simulink model "IEEE30_case"  (R2024b)
settings: Solver=FixedStepAuto  StartTime=0  StopTime=5  FixedStep=1e-7  RelTol=1e-3
values from neighbouring files (symbols this model uses):
  GFL_DFIG_7_C_bus = 0.08    [IEEE30_case_parameters.m]
  GFL_DFIG_7_D_mutual = 2.500000e+3    (= 2500)    [IEEE30_case_parameters.m]
  GFL_DFIG_7_f0 = 60    [IEEE30_case_parameters.m]
  GFL_DFIG_7_gPLLi = 3200    [IEEE30_case_parameters.m]
  GFL_DFIG_7_gPLLp = 650    [IEEE30_case_parameters.m]
  GFL_DFIG_7_H_WT = 0.4    [IEEE30_case_parameters.m]
  GFL_DFIG_7_Hg = 0.8    [IEEE30_case_parameters.m]
  GFL_DFIG_7_Igq_ref = 0    [IEEE30_case_parameters.m]
  GFL_DFIG_7_Ird_ref = 704.45696    [IEEE30_case_parameters.m]
  GFL_DFIG_7_KI_V = -300000    [IEEE30_case_parameters.m]
  GFL_DFIG_7_KP_V = -1000    [IEEE30_case_parameters.m]
  GFL_DFIG_7_Ksh = 1.254300e+4    (= 12543)    [IEEE30_case_parameters.m]
  GFL_DFIG_7_Lg = 0.000483    [IEEE30_case_parameters.m]
  GFL_DFIG_7_Lm_pu = 4    [IEEE30_case_parameters.m]
  GFL_DFIG_7_N = 100    [IEEE30_case_parameters.m]
  GFL_DFIG_7_p = 2    [IEEE30_case_parameters.m]
  GFL_DFIG_7_Pitch = 0    [IEEE30_case_parameters.m]
  GFL_DFIG_7_R = 44    [IEEE30_case_parameters.m]
  GFL_DFIG_7_Rg = 2.000000e-5    (= 2e-05)    [IEEE30_case_parameters.m]
  GFL_DFIG_7_rho = 1.225    [IEEE30_case_parameters.m]
  GFL_DFIG_7_rPLLi = 4500    [IEEE30_case_parameters.m]
  GFL_DFIG_7_rPLLp = 620    [IEEE30_case_parameters.m]
  GFL_DFIG_7_Rs_pu = 0.011    [IEEE30_case_parameters.m]
  GFL_DFIG_7_Sbase = 2.000000e+6    (= 2000000)    [IEEE30_case_parameters.m]
  GFL_DFIG_7_ugq_ref = 0    [IEEE30_case_parameters.m]
  GFL_DFIG_7_usd_ref = 0    [IEEE30_case_parameters.m]
  GFL_DFIG_7_Vbase = 690    [IEEE30_case_parameters.m]
  GFL_DFIG_7_Vdc_ref = 1200    [IEEE30_case_parameters.m]
  GFL_DFIG_7_wind = 12    [IEEE30_case_parameters.m]
  GFL_DFIG_7_wm_ref = 518.184209    [IEEE30_case_parameters.m]
  SG_D_13_D = 0.01056    [IEEE30_case_parameters.m]
  SG_D_13_EnableSaturation = 0    [IEEE30_case_parameters.m]
  SG_D_13_f0 = 60    [IEEE30_case_parameters.m]
  SG_D_13_H = 7.5    [IEEE30_case_parameters.m]
  SG_D_13_K_A = 20    [IEEE30_case_parameters.m]
  SG_D_13_K_E = 1.000000e+1    (= 10)    [IEEE30_case_parameters.m]
  SG_D_13_K_F = 2.363    [IEEE30_case_parameters.m]
  SG_D_13_K_s = 0.5    [IEEE30_case_parameters.m]
  SG_D_13_R_a = 0.001088    [IEEE30_case_parameters.m]
  SG_D_13_S_A = 1    [IEEE30_case_parameters.m]
  SG_D_13_S_B = 0.103    [IEEE30_case_parameters.m]
  SG_D_13_S_N = 10.659857    [IEEE30_case_parameters.m]
  SG_D_13_SpeedPara = 200    [IEEE30_case_parameters.m]
  SG_D_13_T_0 = 0.370163    [IEEE30_case_parameters.m]
  SG_D_13_T_1 = 0.3    [IEEE30_case_parameters.m]
  SG_D_13_T_2 = 0.05    [IEEE30_case_parameters.m]
  SG_D_13_T_3 = 0.02    [IEEE30_case_parameters.m]
  SG_D_13_T_4 = 0.005    [IEEE30_case_parameters.m]
  SG_D_13_T_A = 0.02    [IEEE30_case_parameters.m]
  SG_D_13_T_dd = 8.000000e+0    (= 8)    [IEEE30_case_parameters.m]
  SG_D_13_T_ddd = 0.04    [IEEE30_case_parameters.m]
  SG_D_13_T_E = 0.314    [IEEE30_case_parameters.m]
  SG_D_13_T_F = 0.35    [IEEE30_case_parameters.m]
  SG_D_13_T_qd = 0.8    [IEEE30_case_parameters.m]
  SG_D_13_T_qdd = 0.02    [IEEE30_case_parameters.m]
  SG_D_13_T_speed = 0.1    [IEEE30_case_parameters.m]
  SG_D_13_T_w = 0.5    [IEEE30_case_parameters.m]
  SG_D_13_V_ref = 1.696619    [IEEE30_case_parameters.m]
  SG_D_13_w_ref = 376.991118    [IEEE30_case_parameters.m]
  SG_D_13_x_d = 1.9    [IEEE30_case_parameters.m]
  SG_D_13_x_dd = 0.302    [IEEE30_case_parameters.m]
  SG_D_13_x_ddd = 0.204    [IEEE30_case_parameters.m]
  SG_D_13_x_l = 0.05    [IEEE30_case_parameters.m]
  SG_D_13_x_q = 1.3    [IEEE30_case_parameters.m]
  SG_D_13_x_qd = 0.5    [IEEE30_case_parameters.m]
  SG_D_13_x_qdd = 0.3    [IEEE30_case_parameters.m]
  SG_D_1_D = 0.01056    [IEEE30_case_parameters.m]
  SG_D_1_EnableSaturation = 0    [IEEE30_case_parameters.m]
  SG_D_1_f0 = 60    [IEEE30_case_parameters.m]
  SG_D_1_H = 7.5    [IEEE30_case_parameters.m]
  SG_D_1_K_A = 20    [IEEE30_case_parameters.m]
  SG_D_1_K_E = 1.000000e+1    (= 10)    [IEEE30_case_parameters.m]
  SG_D_1_K_F = 2.363    [IEEE30_case_parameters.m]
  SG_D_1_K_s = 0.5    [IEEE30_case_parameters.m]
  SG_D_1_R_a = 0.001088    [IEEE30_case_parameters.m]
  SG_D_1_S_A = 1    [IEEE30_case_parameters.m]
  SG_D_1_S_B = 0.103    [IEEE30_case_parameters.m]
  SG_D_1_S_N = 10.659857    [IEEE30_case_parameters.m]
  SG_D_1_SpeedPara = 200    [IEEE30_case_parameters.m]
  SG_D_1_T_0 = 0.259812    [IEEE30_case_parameters.m]
  SG_D_1_T_1 = 0.3    [IEEE30_case_parameters.m]
  SG_D_1_T_2 = 0.05    [IEEE30_case_parameters.m]
  SG_D_1_T_3 = 0.02    [IEEE30_case_parameters.m]
  SG_D_1_T_4 = 0.005    [IEEE30_case_parameters.m]
  SG_D_1_T_A = 0.02    [IEEE30_case_parameters.m]
  SG_D_1_T_dd = 8.000000e+0    (= 8)    [IEEE30_case_parameters.m]
  SG_D_1_T_ddd = 0.04    [IEEE30_case_parameters.m]
  SG_D_1_T_E = 0.314    [IEEE30_case_parameters.m]
  SG_D_1_T_F = 0.35    [IEEE30_case_parameters.m]
  SG_D_1_T_qd = 0.8    [IEEE30_case_parameters.m]
  SG_D_1_T_qdd = 0.02    [IEEE30_case_parameters.m]
  SG_D_1_T_speed = 0.1    [IEEE30_case_parameters.m]
  SG_D_1_T_w = 0.5    [IEEE30_case_parameters.m]
  SG_D_1_V_ref = 1.544107    [IEEE30_case_parameters.m]
  SG_D_1_w_ref = 376.991118    [IEEE30_case_parameters.m]
  SG_D_1_x_d = 1.9    [IEEE30_case_parameters.m]
  SG_D_1_x_dd = 0.302    [IEEE30_case_parameters.m]
  SG_D_1_x_ddd = 0.204    [IEEE30_case_parameters.m]
  SG_D_1_x_l = 0.05    [IEEE30_case_parameters.m]
  SG_D_1_x_q = 1.3    [IEEE30_case_parameters.m]
  SG_D_1_x_qd = 0.5    [IEEE30_case_parameters.m]
  SG_D_1_x_qdd = 0.3    [IEEE30_case_parameters.m]
  SG_D_22_D = 0.01056    [IEEE30_case_parameters.m]
  SG_D_22_EnableSaturation = 0    [IEEE30_case_parameters.m]
  SG_D_22_f0 = 60    [IEEE30_case_parameters.m]
  SG_D_22_H = 7.5    [IEEE30_case_parameters.m]
  SG_D_22_K_A = 20    [IEEE30_case_parameters.m]
  SG_D_22_K_E = 1.000000e+1    (= 10)    [IEEE30_case_parameters.m]
  SG_D_22_K_F = 2.363    [IEEE30_case_parameters.m]
  SG_D_22_K_s = 0.5    [IEEE30_case_parameters.m]
  SG_D_22_R_a = 0.001088    [IEEE30_case_parameters.m]
  SG_D_22_S_A = 1    [IEEE30_case_parameters.m]
  SG_D_22_S_B = 0.103    [IEEE30_case_parameters.m]
  SG_D_22_S_N = 10.659857    [IEEE30_case_parameters.m]
  SG_D_22_SpeedPara = 200    [IEEE30_case_parameters.m]
  SG_D_22_T_0 = 0.216121    [IEEE30_case_parameters.m]
  SG_D_22_T_1 = 0.3    [IEEE30_case_parameters.m]
  SG_D_22_T_2 = 0.05    [IEEE30_case_parameters.m]
  SG_D_22_T_3 = 0.02    [IEEE30_case_parameters.m]
  SG_D_22_T_4 = 0.005    [IEEE30_case_parameters.m]
  ... (+126 more)
(part 27 of 27)

== system IEEE30_case/SG_D_27/d_w_SG_D_27_block ==
  note: d_w_SG_D_27 in IEEE30_case
      | $\frac{2\,\pi \,T_{m,\mathrm{SG},D,27}\,f_{0}-D\,\left(w_{\mathrm{SG},D,27}-2\,\pi \,f_{0}\right)+2\,\pi \,f_{0}\,\left(\frac{\psi _{d,\mathrm{SG},D,27}\,\left(\psi _{q,\mathrm{SG},D,27}+\frac{\psi _{\mathrm{gq},\mathrm{SG},D,27}\,\left(x_{l}-x_{\mathrm{qdd}}\right)}{x_{l}-x_{\mathrm{qd}}}+\frac{\psi _{\mathrm{kq},\mathrm{SG},D,27}\,\left(x_{\mathrm{qd}}-x_{\mathrm{qdd}}\right)}{x_{l}-x_{\mathrm{qd}}}\right)}{x_{\mathrm{qdd}}}+\frac{\psi _{q,\mathrm{SG},D,27}\,\left(\frac{\psi _{\mathrm{1d},\mathrm{SG},D,27}\,\left(x_{\mathrm{dd}}-x_{\mathrm{ddd}}\right)}{x_{\mathrm{dd}}-x_{l}}-\psi _{d,\mathrm{SG},D,27}+\frac{\psi _{\mathrm{fd},\mathrm{SG},D,27}\,\left(x_{\mathrm{ddd}}-x_{l}\right)}{x_{\mathrm{dd}}-x_{l}}\right)}{x_{\mathrm{ddd}}}\right)}{2\,H}$
      | Automatically generated on 2025-11-01 18:38:33 .
  State_w_SG_D_27_b6b9b : Inport
  State_T_m_SG_D_27_aac0d : Inport  Port=2
  State_psi_d_SG_D_27_07f9f : Inport  Port=3
  State_psi_gq_SG_D_27_3064d : Inport  Port=4
  State_psi_kq_SG_D_27_cb932 : Inport  Port=5
  State_psi_q_SG_D_27_b32ea : Inport  Port=6
  State_psi_q_SG_D_27_5c8dd : Inport  Port=7
  State_psi_1d_SG_D_27_4e688 : Inport  Port=8
  State_psi_d_SG_D_27_61c40 : Inport  Port=9
  State_psi_fd_SG_D_27_c8345 : Inport  Port=10
  Add_2e8e6 : Sum
  Add_303a9 : Sum
  Add_57abf : Sum
  Add_75058 : Sum
  Add_a1628 : Sum
  Add_acea5 : Sum
  Add_cd7ce : Sum
  Add_f0c45 : Sum
  Constant_-1_29ff5 : Constant  Value=-1
  Constant_-1_34cd9 : Constant  Value=-1
  Constant_-1_56b95 : Constant  Value=-1
  Constant_-1_a6caf : Constant  Value=-1
  Constant_-1_b3e20 : Constant  Value=-1
  Constant_-1_f9b96 : Constant  Value=-1
  Constant_-2.0_76d82 : Constant  Value=-2.0
  Constant_2.0_1f8f8 : Constant  Value=2.0
  Constant_2.0_7f7d3 : Constant  Value=2.0
  Constant_2.0_d4595 : Constant  Value=2.0
  Constant_D_8c3e1 : Constant  Value=D
  Constant_H_ded85 : Constant  Value=H
  Constant_f0_12f10 : Constant  Value=f0
  Constant_f0_4838d : Constant  Value=f0
  Constant_f0_9dd07 : Constant  Value=f0
  Constant_pi_043cd : Constant  Value=pi
  Constant_pi_162ef : Constant  Value=pi
  Constant_pi_f5e6f : Constant  Value=pi
  Constant_x_dd_06dd8 : Constant  Value=x_dd
  Constant_x_dd_b4998 : Constant  Value=x_dd
  Constant_x_dd_e56b0 : Constant  Value=x_dd
  Constant_x_ddd_01a94 : Constant  Value=x_ddd
  Constant_x_ddd_0f3c1 : Constant  Value=x_ddd
  Constant_x_ddd_629a6 : Constant  Value=x_ddd
  Constant_x_l_137ed : Constant  Value=x_l
  Constant_x_l_75ae1 : Constant  Value=x_l
  Constant_x_l_8b67a : Constant  Value=x_l
  Constant_x_l_94bd0 : Constant  Value=x_l
  Constant_x_l_b372a : Constant  Value=x_l
  Constant_x_l_c1f59 : Constant  Value=x_l
  Constant_x_qd_14ded : Constant  Value=x_qd
  Constant_x_qd_7c473 : Constant  Value=x_qd
  Constant_x_qd_95186 : Constant  Value=x_qd
  Constant_x_qdd_94d77 : Constant  Value=x_qdd
  Constant_x_qdd_9e6d3 : Constant  Value=x_qdd
  Constant_x_qdd_b69de : Constant  Value=x_qdd
  Divide_23f65 : Product  Inputs=*/
  Divide_30a31 : Product  Inputs=*/
  Divide_3290f : Product  Inputs=*/
  Divide_3fa4a : Product  Inputs=*/
  Divide_5246f : Product  Inputs=*/
  Divide_75626 : Product  Inputs=*/
  Divide_e346d : Product  Inputs=*/
  Product_04cb2 : Product
  Product_17b45 : Product
  Product_184e9 : Product
  Product_2026d : Product
  Product_23bb4 : Product
  Product_464d9 : Product
  Product_5ac5b : Product
  Product_5bd5d : Product
  Product_68c02 : Product
  Product_8539e : Product
  Product_8a6bf : Product
  Product_90cca : Product
  Product_a0e44 : Product
  Product_a2bd4 : Product
  Product_a4a7d : Product
  Product_aa4b6 : Product
  Product_b2bbd : Product
  Product_cefb1 : Product
  Product_e5ee1 : Product
  Product_e61dc : Product
  Product_e724d : Product
  Product_f112b : Product
  Subtract_1434d : Sum  Inputs=+-
  Subtract_39037 : Sum  Inputs=+-
  Subtract_69b42 : Sum  Inputs=+-
  Subtract_98546 : Sum  Inputs=+-
  Subtract_9c1bb : Sum  Inputs=+-
  Subtract_acd8c : Sum  Inputs=+-
  Subtract_d265d : Sum  Inputs=+-
  Subtract_f7153 : Sum  Inputs=+-
  Blockout_d_w_SG_D_27_0fca4 : Outport
  wires:
  State_psi_q_SG_D_27_5c8dd/1 -> Product_5bd5d/1
  Product_5bd5d/1 -> Divide_75626/1
  Constant_x_l_94bd0/1 -> Product_04cb2/2
  Constant_-1_34cd9/1 -> Product_68c02/1
  Product_68c02/1 -> Add_303a9/1
  Constant_x_l_b372a/1 -> Product_68c02/2
  Subtract_39037/1 -> Product_a0e44/2
  Constant_x_qd_14ded/1 -> Subtract_39037/1
  Constant_2.0_d4595/1 -> Product_cefb1/1
  Constant_x_qdd_9e6d3/1 -> Add_303a9/2
  Product_04cb2/1 -> Add_f0c45/1
  Constant_-1_56b95/1 -> Product_04cb2/1
  Constant_D_8c3e1/1 -> Product_17b45/2
  Constant_x_qdd_94d77/1 -> Subtract_39037/2
  Product_184e9/1 -> Add_a1628/1
  Constant_-1_a6caf/1 -> Product_184e9/1
  Constant_-1_b3e20/1 -> Product_17b45/1
  Constant_x_l_c1f59/1 -> Product_184e9/2
  Product_e724d/1 -> Product_e61dc/1
  Constant_-1_29ff5/1 -> Product_e724d/1
  State_psi_1d_SG_D_27_4e688/1 -> Product_e724d/2
  Subtract_9c1bb/1 -> Product_e61dc/2
  Constant_x_dd_e56b0/1 -> Subtract_9c1bb/1
  Product_a2bd4/1 -> Add_2e8e6/1
  Constant_x_ddd_629a6/1 -> Subtract_9c1bb/2
  Constant_x_l_8b67a/1 -> Subtract_f7153/2
  Product_8539e/1 -> Divide_3290f/1
  State_psi_gq_SG_D_27_3064d/1 -> Product_8539e/1
  Add_303a9/1 -> Product_8539e/2
  Constant_x_qd_95186/1 -> Add_f0c45/2
  Product_a0e44/1 -> Divide_3fa4a/1
  State_psi_kq_SG_D_27_cb932/1 -> Product_a0e44/1
  Constant_x_qd_7c473/1 -> Add_a1628/2
  Subtract_acd8c/1 -> Divide_e346d/2
  Constant_x_dd_06dd8/1 -> Subtract_acd8c/1
  State_w_SG_D_27_b6b9b/1 -> Add_2e8e6/2
  Product_2026d/1 -> Product_b2bbd/1
  Constant_-1_f9b96/1 -> Product_2026d/1
  Constant_x_l_75ae1/1 -> Subtract_acd8c/2
  Subtract_98546/1 -> Product_90cca/2
  Constant_x_ddd_0f3c1/1 -> Subtract_98546/1
  Add_57abf/1 -> Product_b2bbd/2
  Constant_x_l_137ed/1 -> Subtract_98546/2
  Add_f0c45/1 -> Divide_3290f/2
  Add_a1628/1 -> Divide_3fa4a/2
  Product_e61dc/1 -> Divide_e346d/1
  Constant_2.0_7f7d3/1 -> Product_f112b/1
  Product_90cca/1 -> Divide_30a31/1
  State_psi_fd_SG_D_27_c8345/1 -> Product_90cca/1
  Subtract_f7153/1 -> Divide_30a31/2
  Constant_x_dd_b4998/1 -> Subtract_f7153/1
  Constant_pi_f5e6f/1 -> Product_f112b/2
  Divide_3290f/1 -> Subtract_69b42/1
  Divide_3fa4a/1 -> Subtract_69b42/2
  Divide_e346d/1 -> Add_75058/1
  State_psi_d_SG_D_27_61c40/1 -> Add_75058/2
  Constant_-2.0_76d82/1 -> Product_23bb4/1
  Constant_pi_162ef/1 -> Product_23bb4/2
  State_psi_d_SG_D_27_07f9f/1 -> Product_2026d/2
  Subtract_69b42/1 -> Add_57abf/1
  State_psi_q_SG_D_27_b32ea/1 -> Add_57abf/2
  Add_75058/1 -> Subtract_1434d/1
  Divide_30a31/1 -> Subtract_1434d/2
  Product_23bb4/1 -> Product_a2bd4/1
  Add_2e8e6/1 -> Product_a4a7d/2
  Constant_f0_4838d/1 -> Product_a2bd4/2
  Subtract_1434d/1 -> Product_5bd5d/2
  Product_f112b/1 -> Product_464d9/1
  State_T_m_SG_D_27_aac0d/1 -> Product_464d9/2
  Constant_2.0_1f8f8/1 -> Product_8a6bf/1
  Constant_pi_043cd/1 -> Product_8a6bf/2
  Product_b2bbd/1 -> Divide_23f65/1
  Constant_x_qdd_b69de/1 -> Divide_23f65/2
  Constant_x_ddd_01a94/1 -> Divide_75626/2
  Product_17b45/1 -> Product_a4a7d/1
  Product_464d9/1 -> Product_e5ee1/1
  Constant_f0_9dd07/1 -> Product_e5ee1/2
  Product_8a6bf/1 -> Product_aa4b6/1
  Constant_f0_12f10/1 -> Product_aa4b6/2
  Divide_23f65/1 -> Add_cd7ce/1
  Divide_75626/1 -> Add_cd7ce/2
  Product_a4a7d/1 -> Add_acea5/1
  Product_e5ee1/1 -> Add_acea5/2
  Product_aa4b6/1 -> Product_5ac5b/1
  Add_cd7ce/1 -> Product_5ac5b/2
  Add_acea5/1 -> Subtract_d265d/1
  Product_5ac5b/1 -> Subtract_d265d/2
  Constant_H_ded85/1 -> Product_cefb1/2
  Subtract_d265d/1 -> Divide_5246f/1
  Product_cefb1/1 -> Divide_5246f/2
  Divide_5246f/1 -> Blockout_d_w_SG_D_27_0fca4/1

== system IEEE30_case/SG_D_27/i_d_SG_D_27_block ==
  note: i_d_SG_D_27 in IEEE30_case
      | $\frac{\sin\left(\theta _{\mathrm{SG},D,27}\right)\,\left(\frac{\psi _{\mathrm{1d},\mathrm{SG},D,27}\,\left(x_{\mathrm{dd}}-x_{\mathrm{ddd}}\right)}{x_{\mathrm{dd}}-x_{l}}-\psi _{d,\mathrm{SG},D,27}+\frac{\psi _{\mathrm{fd},\mathrm{SG},D,27}\,\left(x_{\mathrm{ddd}}-x_{l}\right)}{x_{\mathrm{dd}}-x_{l}}\right)}{x_{\mathrm{ddd}}}-\frac{\cos\left(\theta _{\mathrm{SG},D,27}\right)\,\left(\psi _{q,\mathrm{SG},D,27}+\frac{\psi _{\mathrm{gq},\mathrm{SG},D,27}\,\left(x_{l}-x_{\mathrm{qdd}}\right)}{x_{l}-x_{\mathrm{qd}}}+\frac{\psi _{\mathrm{kq},\mathrm{SG},D,27}\,\left(x_{\mathrm{qd}}-x_{\mathrm{qdd}}\right)}{x_{l}-x_{\mathrm{qd}}}\right)}{x_{\mathrm{qdd}}}$
      | Automatically generated on 2025-11-01 18:38:54 .
  State_psi_gq_SG_D_27_d72b2 : Inport
  State_psi_kq_SG_D_27_7b606 : Inport  Port=2
  State_psi_q_SG_D_27_720da : Inport  Port=3
  State_theta_SG_D_27_3e79c : Inport  Port=4
  State_psi_1d_SG_D_27_ec66c : Inport  Port=5
  State_psi_d_SG_D_27_2629b : Inport  Port=6
  State_psi_fd_SG_D_27_68d93 : Inport  Port=7
  State_theta_SG_D_27_e4dee : Inport  Port=8
  Add_046e1 : Sum
  Add_48459 : Sum
  Add_4c6cd : Sum
  Add_58a81 : Sum
  Add_a0079 : Sum
  Constant_-1_158e0 : Constant  Value=-1
  Constant_-1_4e743 : Constant  Value=-1
  Constant_-1_5b6ed : Constant  Value=-1
  Constant_-1_c3616 : Constant  Value=-1
  Constant_-1_faaf0 : Constant  Value=-1
  Constant_x_dd_63890 : Constant  Value=x_dd
  Constant_x_dd_6695a : Constant  Value=x_dd
  Constant_x_dd_f632d : Constant  Value=x_dd
  Constant_x_ddd_66939 : Constant  Value=x_ddd
  Constant_x_ddd_98d7e : Constant  Value=x_ddd
  Constant_x_ddd_a84ae : Constant  Value=x_ddd
  Constant_x_l_4ad0e : Constant  Value=x_l
  Constant_x_l_5edd0 : Constant  Value=x_l
  Constant_x_l_6848f : Constant  Value=x_l
  Constant_x_l_94647 : Constant  Value=x_l
  Constant_x_l_a28b2 : Constant  Value=x_l
  Constant_x_l_f2c28 : Constant  Value=x_l
  Constant_x_qd_66f17 : Constant  Value=x_qd
  Constant_x_qd_70e1a : Constant  Value=x_qd
  Constant_x_qd_f060d : Constant  Value=x_qd
  Constant_x_qdd_618e4 : Constant  Value=x_qdd
  Constant_x_qdd_a4c7d : Constant  Value=x_qdd
  Constant_x_qdd_c128c : Constant  Value=x_qdd
  Divide_068a1 : Product  Inputs=*/
  Divide_1de40 : Product  Inputs=*/
  Divide_998e5 : Product  Inputs=*/
  Divide_ae3ac : Product  Inputs=*/
  Divide_b796e : Product  Inputs=*/
  Divide_ff9bd : Product  Inputs=*/
  MathFunc_cos_f1dad : Trigonometry  Operator=cos
  MathFunc_sin_0c135 : Trigonometry
  Product_18ff4 : Product
  Product_42acd : Product
  Product_47d9c : Product
  Product_52983 : Product
  Product_6da0d : Product
  Product_9be3b : Product
  Product_ae6d9 : Product
  Product_b00a7 : Product
  Product_e84f7 : Product
  Product_ebc30 : Product
  Product_ec088 : Product
  Subtract_3a663 : Sum  Inputs=+-
  Subtract_4f03f : Sum  Inputs=+-
  Subtract_4f32f : Sum  Inputs=+-
  Subtract_622b2 : Sum  Inputs=+-
  Subtract_83ac3 : Sum  Inputs=+-
  Subtract_bf048 : Sum  Inputs=+-
  Subtract_c5ede : Sum  Inputs=+-
  Subtract_dd95e : Sum  Inputs=+-
  Blockout_i_d_SG_D_27_44f73 : Outport
  wires:
  Divide_ae3ac/1 -> Subtract_c5ede/2
  Product_ae6d9/1 -> Add_48459/1
  Constant_-1_5b6ed/1 -> Product_ae6d9/1
  Constant_x_l_5edd0/1 -> Product_ebc30/2
  Divide_068a1/1 -> Subtract_c5ede/1
  Constant_-1_faaf0/1 -> Product_18ff4/1
  Product_18ff4/1 -> Add_4c6cd/1
  Constant_x_l_94647/1 -> Product_18ff4/2
  MathFunc_cos_f1dad/1 -> Product_b00a7/2
  Subtract_3a663/1 -> Product_42acd/2
  Constant_x_qd_f060d/1 -> Subtract_3a663/1
  Constant_x_qdd_c128c/1 -> Add_4c6cd/2
  Product_ebc30/1 -> Add_046e1/1
  Constant_-1_4e743/1 -> Product_ebc30/1
  Product_ec088/1 -> Divide_1de40/1
  Constant_x_qdd_618e4/1 -> Subtract_3a663/2
  Constant_x_l_6848f/1 -> Product_ae6d9/2
  Product_6da0d/1 -> Product_9be3b/1
  Constant_-1_c3616/1 -> Product_6da0d/1
  State_psi_gq_SG_D_27_d72b2/1 -> Product_ec088/1
  Add_4c6cd/1 -> Product_ec088/2
  Constant_x_qd_66f17/1 -> Add_046e1/2
  Product_42acd/1 -> Divide_998e5/1
  State_psi_kq_SG_D_27_7b606/1 -> Product_42acd/1
  Add_046e1/1 -> Divide_1de40/2
  Constant_x_qd_70e1a/1 -> Add_48459/2
  State_theta_SG_D_27_3e79c/1 -> MathFunc_cos_f1dad/1
  State_psi_1d_SG_D_27_ec66c/1 -> Product_6da0d/2
  Subtract_dd95e/1 -> Product_9be3b/2
  Constant_x_dd_63890/1 -> Subtract_dd95e/1
  Constant_x_ddd_66939/1 -> Subtract_dd95e/2
  Add_48459/1 -> Divide_998e5/2
  Subtract_bf048/1 -> Divide_b796e/2
  Constant_x_dd_f632d/1 -> Subtract_bf048/1
  Constant_x_l_a28b2/1 -> Subtract_bf048/2
  Subtract_4f03f/1 -> Product_47d9c/2
  Constant_x_ddd_a84ae/1 -> Subtract_4f03f/1
  Constant_x_l_f2c28/1 -> Subtract_4f03f/2
  Subtract_83ac3/1 -> Divide_ff9bd/2
  Constant_x_dd_6695a/1 -> Subtract_83ac3/1
  Divide_1de40/1 -> Subtract_4f32f/1
  Divide_998e5/1 -> Subtract_4f32f/2
  Product_9be3b/1 -> Divide_b796e/1
  Product_47d9c/1 -> Divide_ff9bd/1
  State_psi_fd_SG_D_27_68d93/1 -> Product_47d9c/1
  Constant_x_l_4ad0e/1 -> Subtract_83ac3/2
  Product_e84f7/1 -> Divide_ae3ac/1
  Subtract_4f32f/1 -> Add_58a81/1
  Product_b00a7/1 -> Divide_068a1/1
  Add_58a81/1 -> Product_52983/2
  State_psi_q_SG_D_27_720da/1 -> Add_58a81/2
  Constant_x_qdd_a4c7d/1 -> Divide_068a1/2
  Divide_b796e/1 -> Add_a0079/1
  State_psi_d_SG_D_27_2629b/1 -> Add_a0079/2
  Subtract_622b2/1 -> Product_e84f7/1
  Constant_-1_158e0/1 -> Product_52983/1
  Add_a0079/1 -> Subtract_622b2/1
  Subtract_c5ede/1 -> Blockout_i_d_SG_D_27_44f73/1
  Divide_ff9bd/1 -> Subtract_622b2/2
  MathFunc_sin_0c135/1 -> Product_e84f7/2
  State_theta_SG_D_27_e4dee/1 -> MathFunc_sin_0c135/1
  Product_52983/1 -> Product_b00a7/1
  Constant_x_ddd_98d7e/1 -> Divide_ae3ac/2

== system IEEE30_case/SG_D_27/i_q_SG_D_27_block ==
  note: i_q_SG_D_27 in IEEE30_case
      | $-\frac{\sin\left(\theta _{\mathrm{SG},D,27}\right)\,\left(\psi _{q,\mathrm{SG},D,27}+\frac{\psi _{\mathrm{gq},\mathrm{SG},D,27}\,\left(x_{l}-x_{\mathrm{qdd}}\right)}{x_{l}-x_{\mathrm{qd}}}+\frac{\psi _{\mathrm{kq},\mathrm{SG},D,27}\,\left(x_{\mathrm{qd}}-x_{\mathrm{qdd}}\right)}{x_{l}-x_{\mathrm{qd}}}\right)}{x_{\mathrm{qdd}}}-\frac{\cos\left(\theta _{\mathrm{SG},D,27}\right)\,\left(\frac{\psi _{\mathrm{1d},\mathrm{SG},D,27}\,\left(x_{\mathrm{dd}}-x_{\mathrm{ddd}}\right)}{x_{\mathrm{dd}}-x_{l}}-\psi _{d,\mathrm{SG},D,27}+\frac{\psi _{\mathrm{fd},\mathrm{SG},D,27}\,\left(x_{\mathrm{ddd}}-x_{l}\right)}{x_{\mathrm{dd}}-x_{l}}\right)}{x_{\mathrm{ddd}}}$
      | Automatically generated on 2025-11-01 18:38:59 .
  State_psi_gq_SG_D_27_0dda8 : Inport
  State_psi_kq_SG_D_27_df7da : Inport  Port=2
  State_psi_q_SG_D_27_1d36b : Inport  Port=3
  State_theta_SG_D_27_54b2e : Inport  Port=4
  State_psi_1d_SG_D_27_1a223 : Inport  Port=5
  State_psi_d_SG_D_27_bea5b : Inport  Port=6
  State_psi_fd_SG_D_27_8eaba : Inport  Port=7
  State_theta_SG_D_27_83f88 : Inport  Port=8
  Add_1d676 : Sum
  Add_42dd0 : Sum
  Add_86780 : Sum
  Add_a52a5 : Sum
  Add_a884a : Sum
  Add_b0eb6 : Sum
  Constant_-1_15902 : Constant  Value=-1
  Constant_-1_41db9 : Constant  Value=-1
  Constant_-1_470af : Constant  Value=-1
  Constant_-1_6887f : Constant  Value=-1
  Constant_-1_f42df : Constant  Value=-1
  Constant_x_dd_6af1a : Constant  Value=x_dd
  Constant_x_dd_c43e7 : Constant  Value=x_dd
  Constant_x_dd_ff140 : Constant  Value=x_dd
  Constant_x_ddd_091e5 : Constant  Value=x_ddd
  Constant_x_ddd_a7bbd : Constant  Value=x_ddd
  Constant_x_ddd_b0388 : Constant  Value=x_ddd
  Constant_x_l_29c42 : Constant  Value=x_l
  Constant_x_l_3437c : Constant  Value=x_l
  Constant_x_l_373ed : Constant  Value=x_l
  Constant_x_l_49b0e : Constant  Value=x_l
  Constant_x_l_60322 : Constant  Value=x_l
  Constant_x_l_b8791 : Constant  Value=x_l
  Constant_x_qd_769e0 : Constant  Value=x_qd
  Constant_x_qd_78528 : Constant  Value=x_qd
  Constant_x_qd_e936e : Constant  Value=x_qd
  Constant_x_qdd_2efdb : Constant  Value=x_qdd
  Constant_x_qdd_45695 : Constant  Value=x_qdd
  Constant_x_qdd_710e9 : Constant  Value=x_qdd
  Divide_39af3 : Product  Inputs=*/
  Divide_54641 : Product  Inputs=*/
  Divide_7311f : Product  Inputs=*/
  Divide_970e8 : Product  Inputs=*/
  Divide_be190 : Product  Inputs=*/
  Divide_f2766 : Product  Inputs=*/
  MathFunc_cos_69b84 : Trigonometry  Operator=cos
  MathFunc_sin_17220 : Trigonometry
  Product_0494f : Product
  Product_070ff : Product
  Product_37fc4 : Product
  Product_63fd3 : Product
  Product_7c684 : Product
  Product_9cc5e : Product
  Product_a34ed : Product
  Product_b2b91 : Product
  Product_bc4b5 : Product
  Product_f4379 : Product
  Product_ff288 : Product
  Subtract_04f27 : Sum  Inputs=+-
  Subtract_0b44f : Sum  Inputs=+-
  Subtract_687b6 : Sum  Inputs=+-
  Subtract_999be : Sum  Inputs=+-
  Subtract_cc6eb : Sum  Inputs=+-
  Subtract_dc00c : Sum  Inputs=+-
  Subtract_e714a : Sum  Inputs=+-
  Blockout_i_q_SG_D_27_b805d : Outport
  wires:
  Product_bc4b5/1 -> Add_1d676/1
  Constant_-1_15902/1 -> Product_bc4b5/1
  Subtract_0b44f/1 -> Divide_54641/2
  Constant_x_dd_ff140/1 -> Subtract_0b44f/1
  Constant_-1_f42df/1 -> Product_9cc5e/1
  State_psi_1d_SG_D_27_1a223/1 -> Product_7c684/2
  State_psi_gq_SG_D_27_0dda8/1 -> Product_b2b91/1
  Constant_x_l_3437c/1 -> Product_9cc5e/2
  Constant_x_qdd_710e9/1 -> Add_b0eb6/2
  Product_9cc5e/1 -> Add_b0eb6/1
  Add_86780/1 -> Blockout_i_q_SG_D_27_b805d/1
  Subtract_cc6eb/1 -> Product_070ff/2
  Constant_x_l_b8791/1 -> Product_bc4b5/2
  Constant_x_qd_78528/1 -> Subtract_cc6eb/1
  Constant_x_qdd_45695/1 -> Subtract_cc6eb/2
  Product_a34ed/1 -> Add_a52a5/1
  Constant_-1_41db9/1 -> Product_a34ed/1
  Product_7c684/1 -> Product_37fc4/1
  Constant_-1_470af/1 -> Product_7c684/1
  Constant_x_l_60322/1 -> Product_a34ed/2
  Constant_x_qd_e936e/1 -> Add_a52a5/2
  Add_b0eb6/1 -> Product_b2b91/2
  Divide_970e8/1 -> Subtract_999be/2
  Constant_x_qd_769e0/1 -> Add_1d676/2
  Product_070ff/1 -> Divide_970e8/1
  State_psi_kq_SG_D_27_df7da/1 -> Product_070ff/1
  Constant_x_l_373ed/1 -> Subtract_e714a/2
  Subtract_dc00c/1 -> Product_37fc4/2
  Constant_x_dd_6af1a/1 -> Subtract_dc00c/1
  Constant_x_ddd_a7bbd/1 -> Subtract_687b6/1
  Constant_x_ddd_091e5/1 -> Subtract_dc00c/2
  Product_b2b91/1 -> Divide_39af3/1
  Product_63fd3/1 -> Divide_be190/1
  Add_1d676/1 -> Divide_39af3/2
  Add_a52a5/1 -> Divide_970e8/2
  Subtract_687b6/1 -> Product_f4379/2
  Constant_x_l_49b0e/1 -> Subtract_0b44f/2
  Constant_x_l_29c42/1 -> Subtract_687b6/2
  Divide_39af3/1 -> Subtract_999be/1
  State_psi_q_SG_D_27_1d36b/1 -> Add_a884a/2
  Product_37fc4/1 -> Divide_54641/1
  Constant_-1_6887f/1 -> Product_0494f/1
  State_psi_fd_SG_D_27_8eaba/1 -> Product_f4379/1
  Divide_be190/1 -> Add_86780/1
  Constant_x_dd_c43e7/1 -> Subtract_e714a/1
  Subtract_999be/1 -> Add_a884a/1
  Divide_54641/1 -> Add_42dd0/1
  Divide_f2766/1 -> Subtract_04f27/2
  State_psi_d_SG_D_27_bea5b/1 -> Add_42dd0/2
  Product_f4379/1 -> Divide_f2766/1
  Subtract_e714a/1 -> Divide_f2766/2
  Add_a884a/1 -> Product_0494f/2
  State_theta_SG_D_27_54b2e/1 -> MathFunc_sin_17220/1
  Add_42dd0/1 -> Subtract_04f27/1
  State_theta_SG_D_27_83f88/1 -> MathFunc_cos_69b84/1
  Product_0494f/1 -> Product_63fd3/1
  MathFunc_sin_17220/1 -> Product_63fd3/2
  Subtract_04f27/1 -> Product_ff288/1
  MathFunc_cos_69b84/1 -> Product_ff288/2
  Divide_7311f/1 -> Add_86780/2
  Constant_x_qdd_2efdb/1 -> Divide_be190/2
  Product_ff288/1 -> Divide_7311f/1
  Constant_x_ddd_b0388/1 -> Divide_7311f/2

== system IEEE30_case/SG_D_27/theta_SG_D_27_out_block ==
  note: theta_SG_D_27_out in IEEE30_case
      | $\theta _{\mathrm{SG},D,27}$
      | Automatically generated on 2025-11-01 18:39:04 .
  State_theta_SG_D_27_c2ad6 : Inport
  Blockout_theta_SG_D_27_out_fd4a4 : Outport
  wires:
  State_theta_SG_D_27_c2ad6/1 -> Blockout_theta_SG_D_27_out_fd4a4/1

== system IEEE30_case/SG_D_27/w_SG_D_27_out_block ==
  note: w_SG_D_27_out in IEEE30_case
      | $w_{\mathrm{SG},D,27}$
      | Automatically generated on 2025-11-01 18:39:04 .
  State_w_SG_D_27_8ae81 : Inport
  Blockout_w_SG_D_27_out_337ec : Outport
  wires:
  State_w_SG_D_27_8ae81/1 -> Blockout_w_SG_D_27_out_337ec/1

== system IEEE30_case/Subsystem1/Subsystem ==
  uq : Inport
  ud : Inport  Port=2
  id : Inport  Port=3
  iq : Inport  Port=4
  Add : Sum
  Product : Product
  Product1 : Product
  Out1 : Outport
  wires:
  Product/1 -> Add/1
  id/1 -> Product/2
  ud/1 -> Product/1
  uq/1 -> Product1/1
  Product1/1 -> Add/2
  Add/1 -> Out1/1
  iq/1 -> Product1/2

== system IEEE30_case/Subsystem1/Subsystem1 ==
  id : Inport
  iq : Inport  Port=2
  ud : Inport  Port=3
  uq : Inport  Port=4
  Add1 : Sum  Inputs=+-
  Product : Product
  Product1 : Product
  Out1 : Outport
  wires:
  Product1/1 -> Add1/2
  ud/1 -> Product1/2
  Add1/1 -> Out1/1
  Product/1 -> Add1/1
  iq/1 -> Product1/1
  id/1 -> Product/2
  uq/1 -> Product/1

== system IEEE30_case/Subsystem2/Subsystem ==
  uq : Inport
  ud : Inport  Port=2
  id : Inport  Port=3
  iq : Inport  Port=4
  Add : Sum
  Product : Product
  Product1 : Product
  Out1 : Outport
  wires:
  Product/1 -> Add/1
  id/1 -> Product/2
  ud/1 -> Product/1
  uq/1 -> Product1/1
  Product1/1 -> Add/2
  Add/1 -> Out1/1
  iq/1 -> Product1/2

== system IEEE30_case/Subsystem2/Subsystem1 ==
  id : Inport
  iq : Inport  Port=2
  ud : Inport  Port=3
  uq : Inport  Port=4
  Add1 : Sum  Inputs=+-
  Product : Product
  Product1 : Product
  Out1 : Outport
  wires:
  Product1/1 -> Add1/2
  ud/1 -> Product1/2
  Add1/1 -> Out1/1
  Product/1 -> Add1/1
  iq/1 -> Product1/1
  id/1 -> Product/2
  uq/1 -> Product/1

== system IEEE30_case/Subsystem3/Subsystem ==
  uq : Inport
  ud : Inport  Port=2
  id : Inport  Port=3
  iq : Inport  Port=4
  Add : Sum
  Product : Product
  Product1 : Product
  Out1 : Outport
  wires:
  Product/1 -> Add/1
  id/1 -> Product/2
  ud/1 -> Product/1
  uq/1 -> Product1/1
  Product1/1 -> Add/2
  Add/1 -> Out1/1
  iq/1 -> Product1/2

== system IEEE30_case/Subsystem3/Subsystem1 ==
  id : Inport
  iq : Inport  Port=2
  ud : Inport  Port=3
  uq : Inport  Port=4
  Add1 : Sum  Inputs=+-
  Product : Product
  Product1 : Product
  Out1 : Outport
  wires:
  Product1/1 -> Add1/2
  ud/1 -> Product1/2
  Add1/1 -> Out1/1
  Product/1 -> Add1/1
  iq/1 -> Product1/1
  id/1 -> Product/2
  uq/1 -> Product/1

== system IEEE30_case/Subsystem4/Subsystem ==
  uq : Inport
  ud : Inport  Port=2
  id : Inport  Port=3
  iq : Inport  Port=4
  Add : Sum
  Product : Product
  Product1 : Product
  Out1 : Outport
  wires:
  iq/1 -> Product1/2
  Add/1 -> Out1/1
  Product1/1 -> Add/2
  uq/1 -> Product1/1
  ud/1 -> Product/1
  id/1 -> Product/2
  Product/1 -> Add/1

== system IEEE30_case/Subsystem4/Subsystem1 ==
  id : Inport
  iq : Inport  Port=2
  ud : Inport  Port=3
  uq : Inport  Port=4
  Add1 : Sum  Inputs=+-
  Product : Product
  Product1 : Product
  Out1 : Outport
  wires:
  uq/1 -> Product/1
  id/1 -> Product/2
  iq/1 -> Product1/1
  Product/1 -> Add1/1
  Add1/1 -> Out1/1
  ud/1 -> Product1/2
  Product1/1 -> Add1/2

== system IEEE30_case/Subsystem5/Subsystem ==
  uq : Inport
  ud : Inport  Port=2
  id : Inport  Port=3
  iq : Inport  Port=4
  Add : Sum
  Product : Product
  Product1 : Product
  Out1 : Outport
  wires:
  Product/1 -> Add/1
  id/1 -> Product/2
  ud/1 -> Product/1
  uq/1 -> Product1/1
  Product1/1 -> Add/2
  Add/1 -> Out1/1
  iq/1 -> Product1/2

== system IEEE30_case/Subsystem5/Subsystem1 ==
  id : Inport
  iq : Inport  Port=2
  ud : Inport  Port=3
  uq : Inport  Port=4
  Add1 : Sum  Inputs=+-
  Product : Product
  Product1 : Product
  Out1 : Outport
  wires:
  Product1/1 -> Add1/2
  ud/1 -> Product1/2
  Add1/1 -> Out1/1
  Product/1 -> Add1/1
  iq/1 -> Product1/1
  id/1 -> Product/2
  uq/1 -> Product/1

== system IEEE30_case/Subsystem6/Subsystem ==
  uq : Inport
  ud : Inport  Port=2
  id : Inport  Port=3
  iq : Inport  Port=4
  Add : Sum
  Product : Product
  Product1 : Product
  Out1 : Outport
  wires:
  Product/1 -> Add/1
  id/1 -> Product/2
  ud/1 -> Product/1
  uq/1 -> Product1/1
  Product1/1 -> Add/2
  Add/1 -> Out1/1
  iq/1 -> Product1/2

== system IEEE30_case/Subsystem6/Subsystem1 ==
  id : Inport
  iq : Inport  Port=2
  ud : Inport  Port=3
  uq : Inport  Port=4
  Add1 : Sum  Inputs=+-
  Product : Product
  Product1 : Product
  Out1 : Outport
  wires:
  Product1/1 -> Add1/2
  ud/1 -> Product1/2
  Add1/1 -> Out1/1
  Product/1 -> Add1/1
  iq/1 -> Product1/1
  id/1 -> Product/2
  uq/1 -> Product/1

== system IEEE30_case/Subsystem7/Subsystem ==
  uq : Inport
  ud : Inport  Port=2
  id : Inport  Port=3
  iq : Inport  Port=4
  Add : Sum
  Product : Product
  Product1 : Product
  Out1 : Outport
  wires:
  iq/1 -> Product1/2
  Add/1 -> Out1/1
  Product1/1 -> Add/2
  uq/1 -> Product1/1
  ud/1 -> Product/1
  id/1 -> Product/2
  Product/1 -> Add/1

== system IEEE30_case/Subsystem7/Subsystem1 ==
  id : Inport
  iq : Inport  Port=2
  ud : Inport  Port=3
  uq : Inport  Port=4
  Add1 : Sum  Inputs=+-
  Product : Product
  Product1 : Product
  Out1 : Outport
  wires:
  uq/1 -> Product/1
  id/1 -> Product/2
  iq/1 -> Product1/1
  Product/1 -> Add1/1
  Add1/1 -> Out1/1
  ud/1 -> Product1/2
  Product1/1 -> Add1/2
